simulink model "rtwdemo_fileprocess"  (Simulink 7.6)
settings: Solver=FixedStepDiscrete  StartTime=0.0  StopTime=48  FixedStep=1  RelTol=1e-3
libraries: rtwdemowidgets x2
Description:
  | Custom File Processing Using the Target Language Compiler
settings Model: Creator=The MathWorks Inc.  ParamWorkspaceSource=ReferencedWorkspace  CovMetricSettings=d  ExtModeTrigMode=oneshot  ExtModeArmWhenConnect=off  ExtModeAutoUpdateStatusClock=off
settings MATStruct: SampleTime=1  Offset=0  Priority=[20.0]
settings DataIOCC: LimitDataPoints=off  SaveFormat=StructureWithTime  SaveOutput=off  SaveTime=off  SignalLoggingName=sigsOut
settings OptimizationCC: InlineParams=on  InlineInvariantSignals=on  PassReuseOutputArgsAs=Individual arguments  StateBitsets=on  DataBitsets=on  UseTempVars=on  ZeroExternalMemoryAtStartup=off  ZeroInternalMemoryAtStartup=off  NoFixptDivByZeroProtection=on  EfficientFloat2IntCast=on  EfficientMapNaN2IntZero=off  OptimizeModelRefInitCode=on  LifeSpan=1
settings DebuggingCC: CheckExecutionContextPreStartOutputMsg=on  CheckExecutionContextRuntimeOutputMsg=on  SolverPrmCheckMsg=none  IntegerOverflowMsg=none  StrictBusMsg=ErrorOnBusTreatedAsVector
settings HardwareCC: ProdIntDivRoundTo=Zero  ProdEndianess=LittleEndian  ProdHWDeviceType=Generic->32-bit Embedded Processor  TargetHWDeviceType=Generic->32-bit Embedded Processor
settings ModelReferenceCC: UpdateModelReferenceTargets=IfOutOfDate
settings RTWCC: SystemTargetFile=ert.tlc  TLCOptions=-p0 -aWarnNonSaturatedBlocks=0  TemplateMakefile=ert_default_tmf  Description=Real-Time Workshop Embedded Coder (no auto configuration)  GenerateReport=on  RTWVerbose=off  ProcessScript=ert_make_rtw_hook  IncludeHyperlinkInReport=on  LaunchReport=on
settings CodeAppCC: ForceParamTrailComments=on  IgnoreCustomStorageClasses=off  IgnoreTestpoints=on  SimulinkDataObjDesc=on  CustomSymbolStrGlobalVar=rt$N$M  CustomSymbolStrType=$N$M  CustomSymbolStrFcn=$N$M$F  CustomSymbolStrMacro=$N$M  InsertBlockDesc=on
settings ERTTargetCC: TargetFcnLib=ansi_tfl_tmw.mat  MultiwordLength=2048  GenerateSampleERTMain=on  SupportNonFinite=off  SupportComplex=off  InlinedParameterPlacement=NonHierarchical  ERTCustomFileTemplate=rtwdemofileprocess.tlc  ConvertIfToSwitch=off

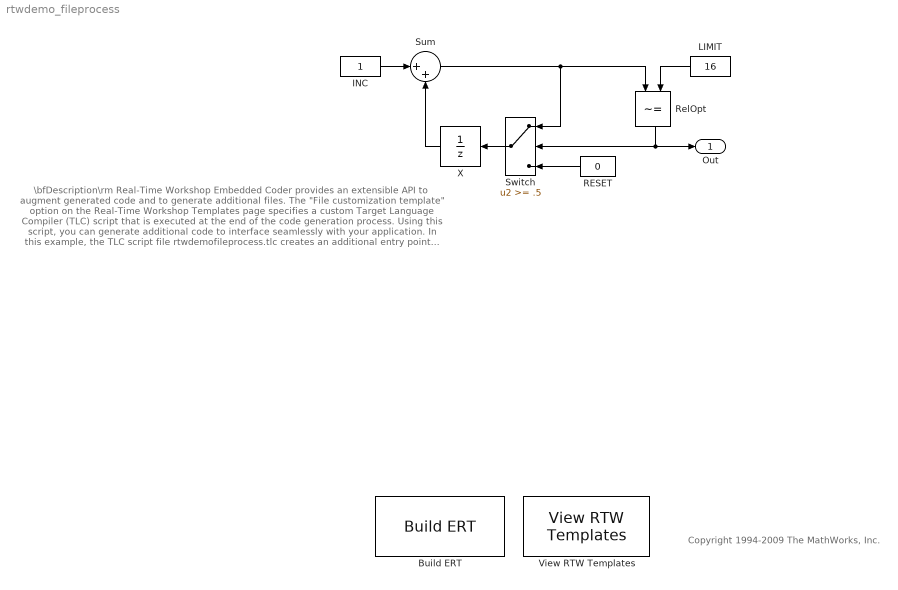
== system rtwdemo_fileprocess ==
  note: \bfDescription\rm
      | Real-Time Workshop Embedded Coder provides an extensible API to augment generated code
      | and to generate additional files.  The "File customization template" option on the Real-Time
      | Workshop Templates page specifies a custom Target Language Compiler (TLC) script that is
      | executed at the end of the code generation process.  Using this script, you can generate additional
      | code to interface seamlessly with your application.
      |
      | In this example, the TLC script file rtwdemofileprocess.tlc creates an additional entry point function,
      | rtwdemo\_fileprocess, to call the step function and initialize the model if necessary.  The initialize
      | function is transparent to the caller.
      |
      | \bfInstructions\rm
      | 1. View the example file process script by double-clicking the yellow button below and clicking the
      |     Edit button to the right of the "File customization template" option.
      | 2. Generate and inspect the code by double-clicking the blue button below.
      | 3. Note that an additional function, rtwdemo\_fileprocess, appears at the end of rtwdemo\_fileprocess.c,
      |     and the entry point is externed in rtwdemo\_fileprocess.h as specified by rtwdemofileprocess.tlc.
  note: Copyright 1994-2009 The MathWorks, Inc.
  Build ERT : rtwdemowidgets/Build ERT  SystemSampleTime=-1  attrib_overrides={'GenerateSampleERTMain','ERTCustomFileTemplate'}
  INC : Constant  OutDataTypeStr=uint8
  LIMIT : Constant  Value=16  OutDataTypeStr=uint8
  RESET : Constant  Value=0  OutDataTypeStr=uint8
  RelOpt : RelationalOperator  Operator=~=  InputSameDT=on
  Sum : Sum  Inputs=|++  InputSameDT=on  OutDataTypeStr=Inherit: Same as first input
  Switch : Switch  Threshold=.5  SaturateOnIntegerOverflow=on  InputSameDT=on
  View RTW Templates : rtwdemowidgets/View RTW Templates  SystemSampleTime=-1
  X : UnitDelay  StateIdentifier=X
  Out : Outport
  wires:
  INC/1 -> Sum/1
  X/1 -> Sum/2
  Switch/1 -> X/1
  Sum/1 -> Switch/1, RelOpt/1
  LIMIT/1 -> RelOpt/2
  RESET/1 -> Switch/3
  RelOpt/1 -> Switch/2, Out/1
